simulink model "WinGEN"  (R2014b)
settings: Solver=ode45  StartTime=0.0  StopTime=10.0  RelTol=1e-3
undefined symbols (not defined in the file): CorrectedWind, Ts
libraries: powerlib_meascontrol x2
settings Model: Creator=amahdizadeh  LastModifiedBy=amahdizadeh

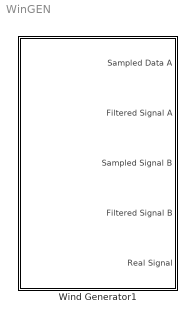
== system WinGEN ==
  Wind Generator1 : Subsystem  AncestorBlock=WT/Wind Generator  mask{WindData=CorrectedWind, Ts_A=.25, Ts_B=.3, PolyOrder=3, Prev_time=.01, Rec_time=6, Ts=Ts}
      mask prompts: WindData "Wind Signal"; Ts_A "Filter A sampling time"; Ts_B "Filter B sampling time"; PolyOrder "Polynimial Order"; Prev_time "Preview Time"; Rec_time "Recording Time"; Ts "Sampling Time"
      mask init:
      | signal = WindData(:,2);
      | time = WindData(:,1);
      | Ts_Org = mean(diff(time));          % original sampling rate
      | 
      | dsRateA = max(fix(Ts_A / Ts_Org),1);
      | dsRateB = max(fix(Ts_B / Ts_Org),1);
      | 
      | %% Filter kernels
      | d0 = lowpass_diff(25,7,0);
      | 
      | %% Aplly the filters
      | %     sig_ds = resample(signal,1,dsRate);  % down sample
      |     sig_dsA = resample(signal,1,dsRateA);  % down sample signal A
      |     sig_dsB = resample(signal,1,dsRateB);  % down sample signal B
      |     % maxflat filters
      | %     y_mf = conv(sig_ds, d1, 'same');     
      |     
      |     y_mfA = conv(sig_dsA, d0, 'same');     
      |     y_mfB = conv(sig_dsB, d0, 'same');     
      |     
      | 
      | %% Generate the output
      | % y = resample(y_mf,dsRate,1);            % up-sample back
      | yA = resample(y_mfA,dsRateA,1);         % up-sample back
      | yB = resample(y_mfB,dsRateB,1);         % up-sample back
      | 
      | % t = linspace(0,time(end),length(y));
      | tA = linspace(0,time(end),length(yA));
      | tB = linspace(0,time(end),length(yB));
      | 
      | % 
      | % org_dt = mean(diff(time));          % original sampling rate
      | % dwn_dt = org_dt*dsRate;             % downsampled rate
      | %Rec_Len = floor(Rec_time/dwn_dt);   % Recording sample no.

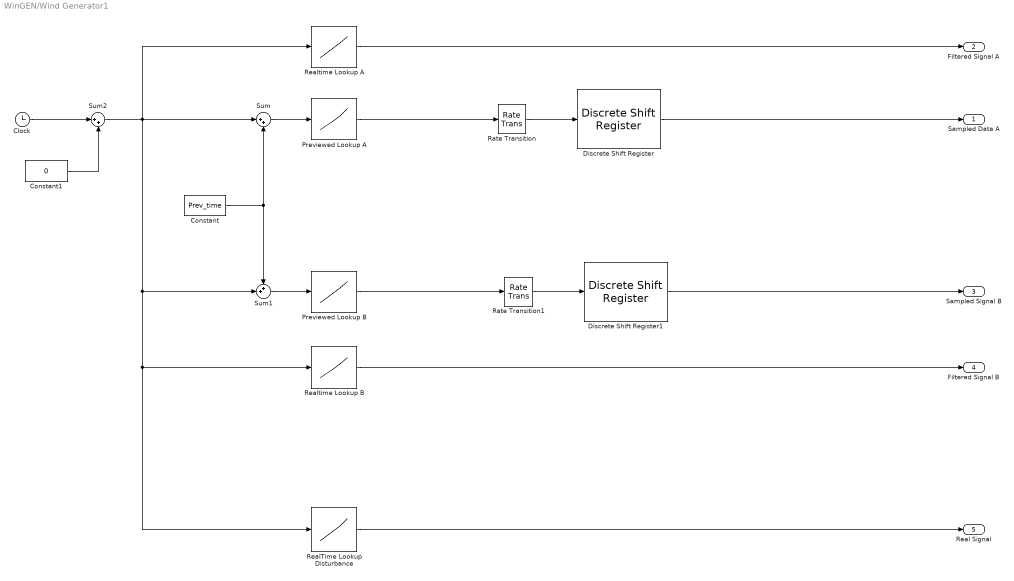
== system WinGEN/Wind Generator1 ==
  Clock : Clock
  Constant : Constant  Value=Prev_time
  Constant1 : Constant  Value=0
  Discrete Shift Register : powerlib_meascontrol/Additional Components/Discrete Shift Register  NSamples=32  InitialValue=0  Ts=50e-6
  Discrete Shift Register1 : powerlib_meascontrol/Additional Components/Discrete Shift Register  NSamples=32  InitialValue=0  Ts=50e-6
  Previewed Lookup A : Lookup_n-D  NumberOfTableDimensions=1  BreakpointsForDimension1=tA  Table=yA  ExtrapMethod=Clip  UseLastTableValue=on  InternalRulePriority=Speed  RndMeth=Simplest  InputSameDT=on
  Previewed Lookup B : Lookup_n-D  NumberOfTableDimensions=1  BreakpointsForDimension1=tB  Table=yB  ExtrapMethod=Clip  UseLastTableValue=on  InternalRulePriority=Speed  RndMeth=Simplest  InputSameDT=on
  Rate Transition : RateTransition  OutPortSampleTime=Ts
  Rate Transition1 : RateTransition  OutPortSampleTime=Ts
  RealTime Lookup Disturbance : Lookup_n-D  NumberOfTableDimensions=1  BreakpointsForDimension1=time  Table=signal  ExtrapMethod=Clip  UseLastTableValue=on  InternalRulePriority=Speed  RndMeth=Simplest  InputSameDT=on
  Realtime Lookup A : Lookup_n-D  NumberOfTableDimensions=1  BreakpointsForDimension1=tA  Table=yA  ExtrapMethod=Clip  UseLastTableValue=on  InternalRulePriority=Speed  RndMeth=Simplest  InputSameDT=on
  Realtime Lookup B : Lookup_n-D  NumberOfTableDimensions=1  BreakpointsForDimension1=tB  Table=yB  ExtrapMethod=Clip  UseLastTableValue=on  InternalRulePriority=Speed  RndMeth=Simplest  InputSameDT=on
  Sum : Sum  Inputs=|++
  Sum1 : Sum  Inputs=++|
  Sum2 : Sum  Inputs=|++
  Sampled Data A : Outport
  Filtered Signal A : Outport  Port=2
  Sampled Signal B : Outport  Port=3
  Filtered Signal B : Outport  Port=4
  Real Signal : Outport  Port=5
  wires:
  Constant1/1 -> Sum2/2
  Clock/1 -> Sum2/1
  Sum2/1 -> Sum/1, Sum1/2, RealTime Lookup Disturbance/1, Realtime Lookup B/1, Realtime Lookup A/1
  Previewed Lookup A/1 -> Rate Transition/1
  RealTime Lookup Disturbance/1 -> Real Signal/1
  Discrete Shift Register/1 -> Sampled Data A/1
  Constant/1 -> Sum/2, Sum1/1
  Sum/1 -> Previewed Lookup A/1
  Rate Transition/1 -> Discrete Shift Register/1
  Sum1/1 -> Previewed Lookup B/1
  Previewed Lookup B/1 -> Rate Transition1/1
  Rate Transition1/1 -> Discrete Shift Register1/1
  Discrete Shift Register1/1 -> Sampled Signal B/1
  Realtime Lookup A/1 -> Filtered Signal A/1
  Realtime Lookup B/1 -> Filtered Signal B/1
